simulink model "cuurent_controlled_circuit"  (R2022a)
settings: Solver=VariableStepAuto  StartTime=0.0  StopTime=25.0  RelTol=1e-3
undefined symbols (not defined in the file or in its folder): DiscIntNeverNeededParam
libraries: fl_lib x82, nesl_utility x65, eeRmsMeasurement x34, eePowerMeasurement x17, ee_lib x16
(part 1 of 3)
settings Model: Creator=qwxt1  LastModifiedBy=qwxt1

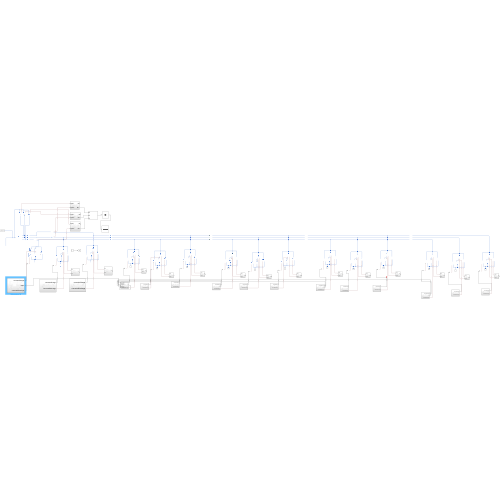
[thumbnail: Simulink's stored preview of the top-level diagram]
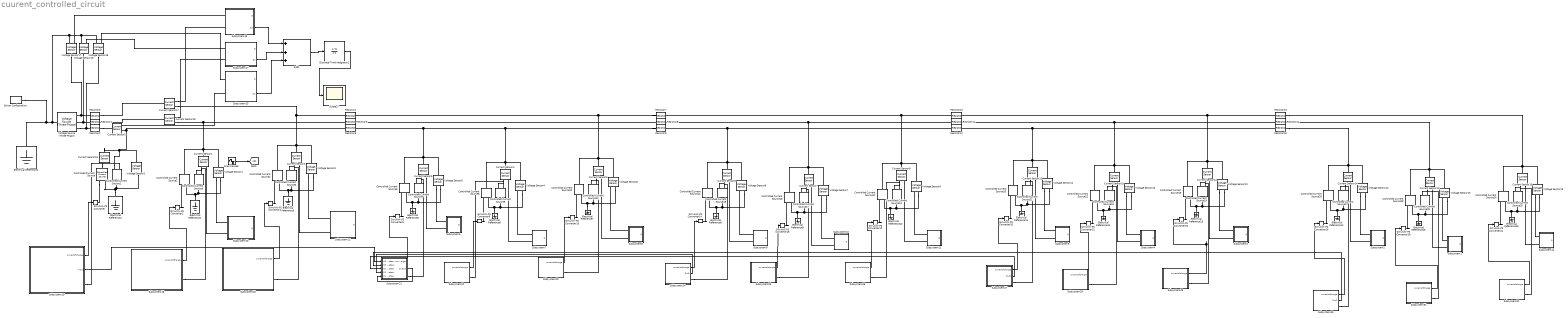
== system cuurent_controlled_circuit ==
  Add1 : Sum  Inputs=+++
  Controlled Current Source{,1..29} (30 alike) : fl_lib/Electrical/Electrical Sources/Controlled Current Source
      settings: SourceProductBaseCode=PW,SS,VE
  Current Sensor{1..17,19} (18 alike) : fl_lib/Electrical/Electrical Sensors/Current Sensor
      settings: SourceProductBaseCode=PW,SS,VE
  Discrete-Time Integrator2 : DiscreteIntegrator  InitialCondition=1500000  ICPrevOutput=DiscIntNeverNeededParam  ICPrevScaledInput=DiscIntNeverNeededParam
  Electrical Reference{1..16} (16 alike) : fl_lib/Electrical/Electrical Elements/Electrical Reference
      settings: SourceProductBaseCode=PW,SS,VE
  Goto : Goto
  Resistor1 : ee_lib/Passive/Resistor  R=0.01989 Ohm  enable_R_tol=0  R_tol=5  tol_distribution=1  nSigma=4  enable_operating_limits=0  operating_limit_action=2  max_working_voltage=100 V  power_rating=1 W  enable_faults=0  fault_action=1  R_faulted=inf Ohm  enable_temporal_fault=0  t_fault=1 s  enable_behavioral_fault=0  max_permissible_current=1 A  t_fail_on_current=1 s  noise_mode=0  sample_time=1e-3 s  repeatability=1  auto_seed=2915145293  user_seed=0  Tdevice=25 degC  power_derating_T1=70 degC  power_derating_T2=155 degC  operating_temperature_range_vec=[-50, 150] degC  alpha=3.93e-3 1/K  Tmeas=25 degC  thermal_mass=100 J/K  temperature_specify=off  temperature_priority=High  temperature=298.15 K  temperature_nominal_specify=off  temperature_nominal_unit=K  temperature_nominal_value=1
  Resistor10 : ee_lib/Passive/Resistor  R=0.040716 Ohm  enable_R_tol=0  R_tol=5  tol_distribution=1  nSigma=4  enable_operating_limits=0  operating_limit_action=2  max_working_voltage=100 V  power_rating=1 W  enable_faults=0  fault_action=1  R_faulted=inf Ohm  enable_temporal_fault=0  t_fault=1 s  enable_behavioral_fault=0  max_permissible_current=1 A  t_fail_on_current=1 s  noise_mode=0  sample_time=1e-3 s  repeatability=1  auto_seed=2513705850  user_seed=0  Tdevice=25 degC  power_derating_T1=70 degC  power_derating_T2=155 degC  operating_temperature_range_vec=[-50, 150] degC  alpha=3.93e-3 1/K  Tmeas=25 degC  thermal_mass=100 J/K  temperature_specify=off  temperature_priority=High  temperature=298.15 K  temperature_nominal_specify=off  temperature_nominal_unit=K  temperature_nominal_value=1
  Resistor11 : ee_lib/Passive/Resistor  R=0.040716 Ohm  enable_R_tol=0  R_tol=5  tol_distribution=1  nSigma=4  enable_operating_limits=0  operating_limit_action=2  max_working_voltage=100 V  power_rating=1 W  enable_faults=0  fault_action=1  R_faulted=inf Ohm  enable_temporal_fault=0  t_fault=1 s  enable_behavioral_fault=0  max_permissible_current=1 A  t_fail_on_current=1 s  noise_mode=0  sample_time=1e-3 s  repeatability=1  auto_seed=961264961  user_seed=0  Tdevice=25 degC  power_derating_T1=70 degC  power_derating_T2=155 degC  operating_temperature_range_vec=[-50, 150] degC  alpha=3.93e-3 1/K  Tmeas=25 degC  thermal_mass=100 J/K  temperature_specify=off  temperature_priority=High  temperature=298.15 K  temperature_nominal_specify=off  temperature_nominal_unit=K  temperature_nominal_value=1
  Resistor12 : ee_lib/Passive/Resistor  R=0.040716 Ohm  enable_R_tol=0  R_tol=5  tol_distribution=1  nSigma=4  enable_operating_limits=0  operating_limit_action=2  max_working_voltage=100 V  power_rating=1 W  enable_faults=0  fault_action=1  R_faulted=inf Ohm  enable_temporal_fault=0  t_fault=1 s  enable_behavioral_fault=0  max_permissible_current=1 A  t_fail_on_current=1 s  noise_mode=0  sample_time=1e-3 s  repeatability=1  auto_seed=3226667450  user_seed=0  Tdevice=25 degC  power_derating_T1=70 degC  power_derating_T2=155 degC  operating_temperature_range_vec=[-50, 150] degC  alpha=3.93e-3 1/K  Tmeas=25 degC  thermal_mass=100 J/K  temperature_specify=off  temperature_priority=High  temperature=298.15 K  temperature_nominal_specify=off  temperature_nominal_unit=K  temperature_nominal_value=1
  Resistor13 : ee_lib/Passive/Resistor  R=0.04524 Ohm  enable_R_tol=0  R_tol=5  tol_distribution=1  nSigma=4  enable_operating_limits=0  operating_limit_action=2  max_working_voltage=100 V  power_rating=1 W  enable_faults=0  fault_action=1  R_faulted=inf Ohm  enable_temporal_fault=0  t_fault=1 s  enable_behavioral_fault=0  max_permissible_current=1 A  t_fail_on_current=1 s  noise_mode=0  sample_time=1e-3 s  repeatability=1  auto_seed=1095625179  user_seed=0  Tdevice=25 degC  power_derating_T1=70 degC  power_derating_T2=155 degC  operating_temperature_range_vec=[-50, 150] degC  alpha=3.93e-3 1/K  Tmeas=25 degC  thermal_mass=100 J/K  temperature_specify=off  temperature_priority=High  temperature=298.15 K  temperature_nominal_specify=off  temperature_nominal_unit=K  temperature_nominal_value=1
  Resistor14 : ee_lib/Passive/Resistor  R=0.04524 Ohm  enable_R_tol=0  R_tol=5  tol_distribution=1  nSigma=4  enable_operating_limits=0  operating_limit_action=2  max_working_voltage=100 V  power_rating=1 W  enable_faults=0  fault_action=1  R_faulted=inf Ohm  enable_temporal_fault=0  t_fault=1 s  enable_behavioral_fault=0  max_permissible_current=1 A  t_fail_on_current=1 s  noise_mode=0  sample_time=1e-3 s  repeatability=1  auto_seed=2173068990  user_seed=0  Tdevice=25 degC  power_derating_T1=70 degC  power_derating_T2=155 degC  operating_temperature_range_vec=[-50, 150] degC  alpha=3.93e-3 1/K  Tmeas=25 degC  thermal_mass=100 J/K  temperature_specify=off  temperature_priority=High  temperature=298.15 K  temperature_nominal_specify=off  temperature_nominal_unit=K  temperature_nominal_value=1
  Resistor15 : ee_lib/Passive/Resistor  R=0.04524 Ohm  enable_R_tol=0  R_tol=5  tol_distribution=1  nSigma=4  enable_operating_limits=0  operating_limit_action=2  max_working_voltage=100 V  power_rating=1 W  enable_faults=0  fault_action=1  R_faulted=inf Ohm  enable_temporal_fault=0  t_fault=1 s  enable_behavioral_fault=0  max_permissible_current=1 A  t_fail_on_current=1 s  noise_mode=0  sample_time=1e-3 s  repeatability=1  auto_seed=3002511661  user_seed=0  Tdevice=25 degC  power_derating_T1=70 degC  power_derating_T2=155 degC  operating_temperature_range_vec=[-50, 150] degC  alpha=3.93e-3 1/K  Tmeas=25 degC  thermal_mass=100 J/K  temperature_specify=off  temperature_priority=High  temperature=298.15 K  temperature_nominal_specify=off  temperature_nominal_unit=K  temperature_nominal_value=1
  Resistor2 : ee_lib/Passive/Resistor  R=0.01989 Ohm  enable_R_tol=0  R_tol=5  tol_distribution=1  nSigma=4  enable_operating_limits=0  operating_limit_action=2  max_working_voltage=100 V  power_rating=1 W  enable_faults=0  fault_action=1  R_faulted=inf Ohm  enable_temporal_fault=0  t_fault=1 s  enable_behavioral_fault=0  max_permissible_current=1 A  t_fail_on_current=1 s  noise_mode=0  sample_time=1e-3 s  repeatability=1  auto_seed=3922919431  user_seed=0  Tdevice=25 degC  power_derating_T1=70 degC  power_derating_T2=155 degC  operating_temperature_range_vec=[-50, 150] degC  alpha=3.93e-3 1/K  Tmeas=25 degC  thermal_mass=100 J/K  temperature_specify=off  temperature_priority=High  temperature=298.15 K  temperature_nominal_specify=off  temperature_nominal_unit=K  temperature_nominal_value=1
  Resistor3 : ee_lib/Passive/Resistor  R=0.01989 Ohm  enable_R_tol=0  R_tol=5  tol_distribution=1  nSigma=4  enable_operating_limits=0  operating_limit_action=2  max_working_voltage=100 V  power_rating=1 W  enable_faults=0  fault_action=1  R_faulted=inf Ohm  enable_temporal_fault=0  t_fault=1 s  enable_behavioral_fault=0  max_permissible_current=1 A  t_fail_on_current=1 s  noise_mode=0  sample_time=1e-3 s  repeatability=1  auto_seed=198304613  user_seed=0  Tdevice=25 degC  power_derating_T1=70 degC  power_derating_T2=155 degC  operating_temperature_range_vec=[-50, 150] degC  alpha=3.93e-3 1/K  Tmeas=25 degC  thermal_mass=100 J/K  temperature_specify=off  temperature_priority=High  temperature=298.15 K  temperature_nominal_specify=off  temperature_nominal_unit=K  temperature_nominal_value=1
  Resistor4 : ee_lib/Passive/Resistor  R=0.0459 Ohm  enable_R_tol=0  R_tol=5  tol_distribution=1  nSigma=4  enable_operating_limits=0  operating_limit_action=2  max_working_voltage=100 V  power_rating=1 W  enable_faults=0  fault_action=1  R_faulted=inf Ohm  enable_temporal_fault=0  t_fault=1 s  enable_behavioral_fault=0  max_permissible_current=1 A  t_fail_on_current=1 s  noise_mode=0  sample_time=1e-3 s  repeatability=1  auto_seed=2813624503  user_seed=0  Tdevice=25 degC  power_derating_T1=70 degC  power_derating_T2=155 degC  operating_temperature_range_vec=[-50, 150] degC  alpha=3.93e-3 1/K  Tmeas=25 degC  thermal_mass=100 J/K  temperature_specify=off  temperature_priority=High  temperature=298.15 K  temperature_nominal_specify=off  temperature_nominal_unit=K  temperature_nominal_value=1
  Resistor5 : ee_lib/Passive/Resistor  R=0.0459 Ohm  enable_R_tol=0  R_tol=5  tol_distribution=1  nSigma=4  enable_operating_limits=0  operating_limit_action=2  max_working_voltage=100 V  power_rating=1 W  enable_faults=0  fault_action=1  R_faulted=inf Ohm  enable_temporal_fault=0  t_fault=1 s  enable_behavioral_fault=0  max_permissible_current=1 A  t_fail_on_current=1 s  noise_mode=0  sample_time=1e-3 s  repeatability=1  auto_seed=698412085  user_seed=0  Tdevice=25 degC  power_derating_T1=70 degC  power_derating_T2=155 degC  operating_temperature_range_vec=[-50, 150] degC  alpha=3.93e-3 1/K  Tmeas=25 degC  thermal_mass=100 J/K  temperature_specify=off  temperature_priority=High  temperature=298.15 K  temperature_nominal_specify=off  temperature_nominal_unit=K  temperature_nominal_value=1
  Resistor6 : ee_lib/Passive/Resistor  R=0.0459 Ohm  enable_R_tol=0  R_tol=5  tol_distribution=1  nSigma=4  enable_operating_limits=0  operating_limit_action=2  max_working_voltage=100 V  power_rating=1 W  enable_faults=0  fault_action=1  R_faulted=inf Ohm  enable_temporal_fault=0  t_fault=1 s  enable_behavioral_fault=0  max_permissible_current=1 A  t_fail_on_current=1 s  noise_mode=0  sample_time=1e-3 s  repeatability=1  auto_seed=511091151  user_seed=0  Tdevice=25 degC  power_derating_T1=70 degC  power_derating_T2=155 degC  operating_temperature_range_vec=[-50, 150] degC  alpha=3.93e-3 1/K  Tmeas=25 degC  thermal_mass=100 J/K  temperature_specify=off  temperature_priority=High  temperature=298.15 K  temperature_nominal_specify=off  temperature_nominal_unit=K  temperature_nominal_value=1
  Resistor7 : ee_lib/Passive/Resistor  R=0.039585 Ohm  enable_R_tol=0  R_tol=5  tol_distribution=1  nSigma=4  enable_operating_limits=0  operating_limit_action=2  max_working_voltage=100 V  power_rating=1 W  enable_faults=0  fault_action=1  R_faulted=inf Ohm  enable_temporal_fault=0  t_fault=1 s  enable_behavioral_fault=0  max_permissible_current=1 A  t_fail_on_current=1 s  noise_mode=0  sample_time=1e-3 s  repeatability=1  auto_seed=2140457305  user_seed=0  Tdevice=25 degC  power_derating_T1=70 degC  power_derating_T2=155 degC  operating_temperature_range_vec=[-50, 150] degC  alpha=3.93e-3 1/K  Tmeas=25 degC  thermal_mass=100 J/K  temperature_specify=off  temperature_priority=High  temperature=298.15 K  temperature_nominal_specify=off  temperature_nominal_unit=K  temperature_nominal_value=1
  Resistor8 : ee_lib/Passive/Resistor  R=0.039585 Ohm  enable_R_tol=0  R_tol=5  tol_distribution=1  nSigma=4  enable_operating_limits=0  operating_limit_action=2  max_working_voltage=100 V  power_rating=1 W  enable_faults=0  fault_action=1  R_faulted=inf Ohm  enable_temporal_fault=0  t_fault=1 s  enable_behavioral_fault=0  max_permissible_current=1 A  t_fail_on_current=1 s  noise_mode=0  sample_time=1e-3 s  repeatability=1  auto_seed=4122068914  user_seed=0  Tdevice=25 degC  power_derating_T1=70 degC  power_derating_T2=155 degC  operating_temperature_range_vec=[-50, 150] degC  alpha=3.93e-3 1/K  Tmeas=25 degC  thermal_mass=100 J/K  temperature_specify=off  temperature_priority=High  temperature=298.15 K  temperature_nominal_specify=off  temperature_nominal_unit=K  temperature_nominal_value=1
  Resistor9 : ee_lib/Passive/Resistor  R=0.039585 Ohm  enable_R_tol=0  R_tol=5  tol_distribution=1  nSigma=4  enable_operating_limits=0  operating_limit_action=2  max_working_voltage=100 V  power_rating=1 W  enable_faults=0  fault_action=1  R_faulted=inf Ohm  enable_temporal_fault=0  t_fault=1 s  enable_behavioral_fault=0  max_permissible_current=1 A  t_fail_on_current=1 s  noise_mode=0  sample_time=1e-3 s  repeatability=1  auto_seed=1461945564  user_seed=0  Tdevice=25 degC  power_derating_T1=70 degC  power_derating_T2=155 degC  operating_temperature_range_vec=[-50, 150] degC  alpha=3.93e-3 1/K  Tmeas=25 degC  thermal_mass=100 J/K  temperature_specify=off  temperature_priority=High  temperature=298.15 K  temperature_nominal_specify=off  temperature_nominal_unit=K  temperature_nominal_value=1
  Scope27 : Scope
  Simulink-PS Converter{,2,4,6,8,10,12,14,16,18,20,22,24,26,28} (15 alike) : nesl_utility/Simulink-PS Converter  PhysicalDomain=network_engine_domain  SubClassName=ps_input  LeftPortType=input  RightPortType=output  PseudoPeriodic=off  Frequencies=[]  NoiseDistribution=none  NoiseParameters=[]  Unit=1  AffineConversion=off  FilteringAndDerivatives=provide  SimscapeFilterOrder=1  InputFilterTimeConstant=0.001  UdotUserProvided=0
      settings: SourceProductBaseCode=SS,PW,VE
  Sine Wave16 : Sin  Frequency=314.6  SampleTime=0
  Solver Configuration : nesl_utility/Solver Configuration  PhysicalDomain=network_engine_domain  SubClassName=solver  LeftPortType=input  RightPortType=generic  Tones=[]  Harmonics=[]  SimulateNoise=off  Profile=off  UseLocalSampling=off  EnableSwitchedLinearOptims=on  FrequencyDomain=off  UseCCode=off  RelTol=0.001  AbsTol=0.001  MinStep=1e-09  ToWorkspace=off  RevertToSquareIcSolve=off  NumHomotopyIterations=100  PhasorMode=off  PhasorModeNumHarmonics=1  IndexReductionMethod=DerivativeReplacement  DoDC=off  ResidualTolerance=1e-09  UseLocalSolver=off  LocalSolverChoice=NE_BACKWARD_EULER_ADVANCER  LocalSolverSampleTime=0.001  DoFixedCost=off  MaxNonlinIter=3  MaxModeIter=2  ComputeImpulses=off  ImpulseIterations=2  LinearAlgebra=auto  LinearAlgebraNumThread=0  EquationFormulation=NE_TIME_EF  DelaysMemoryBudget=1024  AutomaticFiltering=on  FilteringTimeConstant=0.001  PartitionStorageMethod=AS_NEEDED  PartitionMemoryBudget=1024  PartitionMethod=ROBUST
      settings: SourceProductBaseCode=SS,PW,VE
  Subsystem1 : Subsystem
  Subsystem10 : Subsystem
  Subsystem11 : Subsystem
  Subsystem12 : Subsystem
  Subsystem13 : Subsystem
  Subsystem14 : Subsystem
  Subsystem15 : Subsystem
  Subsystem16 : Subsystem
  Subsystem17 : Subsystem
  Subsystem18 : Subsystem
  Subsystem19 : Subsystem
  Subsystem2 : Subsystem
  Subsystem20 : Subsystem
  Subsystem21 : Subsystem
  Subsystem22 : Subsystem
  Subsystem23 : Subsystem
  Subsystem24 : Subsystem
  Subsystem25 : Subsystem
  Subsystem26 : Subsystem
  Subsystem27 : Subsystem
  Subsystem28 : Subsystem
  Subsystem29 : Subsystem
  Subsystem3 : Subsystem
  Subsystem30 : Subsystem
  Subsystem31 : Subsystem
  Subsystem32 : Subsystem
  Subsystem4 : Subsystem
  Subsystem5 : Subsystem
  Subsystem6 : Subsystem
  Subsystem7 : Subsystem
  Subsystem8 : Subsystem
  Subsystem9 : Subsystem
  Voltage Source (Three-Phase) : ee_lib/Sources/Voltage Source (Three-Phase)  vline_rms=400 V  shift=0 deg  freq=50 Hz  impedance_option=0  SShortCircuit=1e6 A*V  XR=15  R=0.01 Ohm  L=3.97e-4 H  harmonic_option=0  harmonic_orders=[5, 7, 11, 13]  harmonic_ratios=[.1, .1, .1, .1]  G_parasitic=0 1/Ohm  I_specify=off  I_priority=None  I=[0, 0, 0] A  I_nominal_specify=off  I_nominal_unit=A  I_nominal_value=1
      settings: SourceProductBaseCode=PS  InternalSimscapePortConfiguration="{\"Bottom\":[],\"Left\":[{\"id\":\"n\",\"label\":\"n\",\"type\":\"foundation.electrical.electrical\"}],\"Right\":[{\"id\":\"a\",\"label\":\"a\",\"type\":\"foundation.electrical.electrical\"},{\"id\":\"b\",\"label\":\"b\",\"type\":\"foundation.electrical.electrical\"},{\"id\":\"c\",\"label\":\"c\",\"type\":\"foundation.electrical.electrical\"}],\"Top\":[]}"
  Voltage Sensor{1..18} (18 alike) : fl_lib/Electrical/Electrical Sensors/Voltage Sensor
      settings: SourceProductBaseCode=PW,SS,VE
  wires:
  Subsystem28/1(currentofcharge) -> Simulink-PS Converter22/1
  Subsystem26/1(currentofcharge) -> Simulink-PS Converter12/1
  Subsystem24/1(currentofcharge) -> Simulink-PS Converter14/1
  Sine Wave16/1 -> Goto/1
  Add1/1 -> Discrete-Time Integrator2/1
  Discrete-Time Integrator2/1 -> Scope27/1
  Subsystem18/2(Q1) -> Add1/1
  Subsystem17/2(Q1) -> Add1/2
  Subsystem15/2(Q1) -> Add1/3
  Subsystem19/1(currentofcharge) -> Simulink-PS Converter/1
  Subsystem20/1(currentofcharge) -> Simulink-PS Converter4/1
  Subsystem30/1(currentofcharge) -> Simulink-PS Converter26/1
  Subsystem21/1(currentofcharge) -> Simulink-PS Converter6/1
  Subsystem22/1(currentofcharge) -> Simulink-PS Converter8/1
  Subsystem23/1(currentofcharge) -> Simulink-PS Converter10/1
  Subsystem25/1(currentofcharge) -> Simulink-PS Converter16/1
  Subsystem27/1(currentofcharge) -> Simulink-PS Converter20/1
  Subsystem29/1(currentofcharge) -> Simulink-PS Converter18/1
  Subsystem31/1(currentofcharge) -> Simulink-PS Converter28/1
  Subsystem32/1(currentofcharge) -> Simulink-PS Converter24/1
  Subsystem16/1(currentofcharge) -> Simulink-PS Converter2/1
  Subsystem19/2(Input) -> Subsystem21/1(M5 Battery)
  Subsystem24/2(Out2) -> Subsystem21/4(M2 Battery)
  Subsystem27/2(Out2) -> Subsystem21/3(M1 Battery)
  Subsystem30/2(Out2) -> Subsystem21/2(M3 Battery)
  Subsystem21/2(Output) -> Subsystem21/5(M4 Battery)
  connections:
  Resistor3/LConn1 -- Voltage Sensor17/LConn1 -- Voltage Source (Three-Phase)/RConn1
  Resistor1/LConn1 -- Voltage Sensor16/LConn1 -- Voltage Source (Three-Phase)/RConn2
  Voltage Source (Three-Phase)/RConn3 -- Voltage Sensor18/LConn1 -- Resistor2/LConn1
  Voltage Sensor3/LConn1 -- Current Sensor17/RConn2 -- Resistor4/LConn1 -- Current Sensor3/LConn1 -- Controlled Current Source4/LConn1
  Resistor6/LConn1 -- Controlled Current Source1/RConn2 -- Current Sensor16/LConn1 -- Voltage Sensor2/LConn1 -- Current Sensor2/RConn2
  Subsystem15/LConn2 -- Current Sensor2/RConn1
  Voltage Sensor1/LConn1 -- Resistor5/LConn1 -- Current Sensor19/RConn2 -- Current Sensor1/LConn1 -- Controlled Current Source2/LConn1
  Electrical Reference4/LConn1 -- Voltage Sensor18/RConn2 -- Voltage Sensor16/RConn2 -- Voltage Sensor17/RConn2 -- Voltage Source (Three-Phase)/LConn1 -- Solver Configuration/RConn1
  Voltage Sensor9/LConn1 -- Resistor10/LConn1 -- Resistor7/RConn1 -- Current Sensor9/LConn1 -- Controlled Current Source12/LConn1
  Resistor8/LConn1 -- Resistor5/RConn1
  Voltage Sensor8/LConn1 -- Resistor12/LConn1 -- Resistor9/RConn1 -- Current Sensor8/LConn1 -- Controlled Current Source14/LConn1
  Voltage Sensor6/LConn1 -- Resistor7/LConn1 -- Resistor4/RConn1 -- Current Sensor6/LConn1 -- Controlled Current Source10/LConn1
  Voltage Sensor7/LConn1 -- Resistor11/LConn1 -- Resistor8/RConn1 -- Current Sensor7/LConn1 -- Controlled Current Source16/LConn1
  Voltage Sensor4/LConn1 -- Resistor9/LConn1 -- Voltage Sensor5/LConn1 -- Current Sensor5/LConn1 -- Controlled Current Source6/LConn1 -- Resistor6/RConn1 -- Current Sensor4/LConn1 -- Controlled Current Source8/LConn1
  Voltage Sensor12/LConn1 -- Resistor13/LConn1 -- Resistor10/RConn1 -- Current Sensor12/LConn1 -- Controlled Current Source18/LConn1
  Voltage Sensor10/LConn1 -- Resistor14/LConn1 -- Resistor11/RConn1 -- Current Sensor10/LConn1 -- Controlled Current Source22/LConn1
  Voltage Sensor11/LConn1 -- Resistor15/LConn1 -- Resistor12/RConn1 -- Current Sensor11/LConn1 -- Controlled Current Source20/LConn1
  Electrical Reference2/LConn1 -- Controlled Current Source2/RConn2 -- Voltage Sensor1/RConn2 -- Controlled Current Source3/LConn1
  Voltage Sensor1/RConn1 -- Subsystem13/LConn1
  Simulink-PS Converter2/RConn1 -- Controlled Current Source2/RConn1
  Current Sensor1/RConn1 -- Subsystem13/LConn2
  Current Sensor1/RConn2 -- Controlled Current Source3/RConn2
  Electrical Reference3/LConn1 -- Controlled Current Source4/RConn2 -- Voltage Sensor3/RConn2 -- Controlled Current Source5/LConn1
  Voltage Sensor3/RConn1 -- Subsystem12/LConn1
  Simulink-PS Converter4/RConn1 -- Controlled Current Source4/RConn1
  Current Sensor3/RConn1 -- Subsystem12/LConn2
  Current Sensor3/RConn2 -- Controlled Current Source5/RConn2
  Electrical Reference6/LConn1 -- Voltage Sensor4/RConn2 -- Controlled Current Source9/LConn1 -- Controlled Current Source8/RConn2
  Electrical Reference7/LConn1 -- Voltage Sensor6/RConn2 -- Controlled Current Source11/LConn1 -- Controlled Current Source10/RConn2
  Electrical Reference5/LConn1 -- Voltage Sensor5/RConn2 -- Controlled Current Source7/LConn1 -- Controlled Current Source6/RConn2
  Simulink-PS Converter6/RConn1 -- Controlled Current Source6/RConn1
  Simulink-PS Converter8/RConn1 -- Controlled Current Source8/RConn1
  Subsystem8/LConn2 -- Current Sensor6/RConn1
  Current Sensor4/RConn2 -- Controlled Current Source9/RConn2
  Subsystem7/LConn1 -- Voltage Sensor4/RConn1
  Current Sensor6/RConn2 -- Controlled Current Source11/RConn2
  Subsystem8/LConn1 -- Voltage Sensor6/RConn1
  Simulink-PS Converter10/RConn1 -- Controlled Current Source10/RConn1
  Current Sensor5/RConn1 -- Subsystem6/LConn2
  Subsystem7/LConn2 -- Current Sensor4/RConn1
  Current Sensor5/RConn2 -- Controlled Current Source7/RConn2
  Controlled Current Source15/LConn1 -- Voltage Sensor8/RConn2 -- Controlled Current Source14/RConn2 -- Electrical Reference8/LConn1
  Controlled Current Source13/LConn1 -- Voltage Sensor9/RConn2 -- Controlled Current Source12/RConn2 -- Electrical Reference10/LConn1
  Controlled Current Source17/LConn1 -- Voltage Sensor7/RConn2 -- Controlled Current Source16/RConn2 -- Electrical Reference9/LConn1
  Simulink-PS Converter12/RConn1 -- Controlled Current Source12/RConn1
  Current Sensor9/RConn2 -- Controlled Current Source13/RConn2
  Simulink-PS Converter16/RConn1 -- Controlled Current Source16/RConn1
  Subsystem9/LConn1 -- Voltage Sensor8/RConn1
  Subsystem11/LConn2 -- Current Sensor9/RConn1
  Current Sensor7/RConn2 -- Controlled Current Source17/RConn2
  Subsystem10/LConn1 -- Voltage Sensor7/RConn1
  Subsystem10/LConn2 -- Current Sensor7/RConn1
  Subsystem9/LConn2 -- Current Sensor8/RConn1
  Current Sensor8/RConn2 -- Controlled Current Source15/RConn2
  Simulink-PS Converter14/RConn1 -- Controlled Current Source14/RConn1
  Subsystem11/LConn1 -- Voltage Sensor9/RConn1
  Controlled Current Source21/LConn1 -- Voltage Sensor11/RConn2 -- Controlled Current Source20/RConn2 -- Electrical Reference11/LConn1
  Controlled Current Source19/LConn1 -- Voltage Sensor12/RConn2 -- Controlled Current Source18/RConn2 -- Electrical Reference13/LConn1
  Controlled Current Source23/LConn1 -- Voltage Sensor10/RConn2 -- Controlled Current Source22/RConn2 -- Electrical Reference12/LConn1
  Simulink-PS Converter18/RConn1 -- Controlled Current Source18/RConn1
  Current Sensor12/RConn2 -- Controlled Current Source19/RConn2
  Simulink-PS Converter22/RConn1 -- Controlled Current Source22/RConn1
  Voltage Sensor11/RConn1 -- Subsystem5/LConn1
  Current Sensor12/RConn1 -- Subsystem3/LConn2
  Current Sensor10/RConn2 -- Controlled Current Source23/RConn2
  Voltage Sensor10/RConn1 -- Subsystem4/LConn1
  Current Sensor10/RConn1 -- Subsystem4/LConn2
  Current Sensor11/RConn1 -- Subsystem5/LConn2
  Current Sensor11/RConn2 -- Controlled Current Source21/RConn2
  Simulink-PS Converter20/RConn1 -- Controlled Current Source20/RConn1
  Voltage Sensor12/RConn1 -- Subsystem3/LConn1
  Voltage Sensor13/LConn1 -- Resistor14/RConn1 -- Current Sensor13/LConn1 -- Controlled Current Source28/LConn1
  Controlled Current Source27/LConn1 -- Voltage Sensor14/RConn2 -- Controlled Current Source26/RConn2 -- Electrical Reference14/LConn1
  Controlled Current Source25/LConn1 -- Voltage Sensor15/RConn2 -- Controlled Current Source24/RConn2 -- Electrical Reference16/LConn1
  Controlled Current Source29/LConn1 -- Voltage Sensor13/RConn2 -- Controlled Current Source28/RConn2 -- Electrical Reference15/LConn1
  Voltage Sensor15/LConn1 -- Resistor13/RConn1 -- Current Sensor15/LConn1 -- Controlled Current Source24/LConn1
  Voltage Sensor14/LConn1 -- Resistor15/RConn1 -- Current Sensor14/LConn1 -- Controlled Current Source26/LConn1
  Simulink-PS Converter24/RConn1 -- Controlled Current Source24/RConn1
  Current Sensor15/RConn2 -- Controlled Current Source25/RConn2
  Simulink-PS Converter28/RConn1 -- Controlled Current Source28/RConn1
  Voltage Sensor14/RConn1 -- Subsystem2/LConn1
  Current Sensor15/RConn1 -- Subsystem14/LConn2
  Current Sensor13/RConn2 -- Controlled Current Source29/RConn2
  Subsystem1/LConn1 -- Voltage Sensor13/RConn1
  Subsystem1/LConn2 -- Current Sensor13/RConn1
  Current Sensor14/RConn1 -- Subsystem2/LConn2
  Current Sensor14/RConn2 -- Controlled Current Source27/RConn2
  Simulink-PS Converter26/RConn1 -- Controlled Current Source26/RConn1
  Voltage Sensor15/RConn1 -- Subsystem14/LConn1
  Current Sensor16/RConn2 -- Controlled Current Source/LConn1
  Controlled Current Source/RConn1 -- Simulink-PS Converter/RConn1
  Resistor2/RConn1 -- Current Sensor2/LConn1
  Voltage Sensor5/RConn1 -- Subsystem6/LConn1
  Electrical Reference1/LConn1 -- Controlled Current Source/RConn2 -- Voltage Sensor2/RConn2 -- Controlled Current Source1/LConn1
  Resistor1/RConn1 -- Current Sensor19/LConn1
  Resistor3/RConn1 -- Current Sensor17/LConn1
  Current Sensor19/RConn1 -- Subsystem17/LConn2
  Current Sensor17/RConn1 -- Subsystem18/LConn2
  Voltage Sensor17/RConn1 -- Subsystem18/LConn1
  Voltage Sensor18/RConn1 -- Subsystem15/LConn1
  Voltage Sensor16/RConn1 -- Subsystem17/LConn1
  Subsystem19/RConn1 -- Controlled Current Source1/RConn1
  Subsystem20/RConn1 -- Controlled Current Source5/RConn1
  Subsystem30/RConn1 -- Controlled Current Source27/RConn1
  Subsystem21/RConn1 -- Controlled Current Source7/RConn1
  Subsystem23/RConn1 -- Controlled Current Source11/RConn1
  Subsystem24/RConn1 -- Controlled Current Source15/RConn1
  Subsystem25/RConn1 -- Controlled Current Source17/RConn1
  Subsystem26/RConn1 -- Controlled Current Source13/RConn1
  Subsystem27/RConn1 -- Controlled Current Source21/RConn1
  Subsystem28/RConn1 -- Controlled Current Source23/RConn1
  Subsystem29/RConn1 -- Controlled Current Source19/RConn1
  Subsystem31/RConn1 -- Controlled Current Source29/RConn1
  Subsystem32/RConn1 -- Controlled Current Source25/RConn1
  Subsystem16/RConn1 -- Controlled Current Source3/RConn1
  Subsystem22/RConn1 -- Controlled Current Source9/RConn1

== system cuurent_controlled_circuit/Subsystem1 ==
  Display3 : Display
  Display4 : Display
  Display5 : Display
  PS-Simulink Converter2 : nesl_utility/PS-Simulink Converter  PhysicalDomain=network_engine_domain  SubClassName=ps_output  LeftPortType=input  RightPortType=output  PseudoPeriodic=off  Frequencies=[]  VectorFormat=inherit  Unit=inherit  AffineConversion=off
      settings: SourceProductBaseCode=SS,PW,VE
  PS-Simulink Converter3 : nesl_utility/PS-Simulink Converter  PhysicalDomain=network_engine_domain  SubClassName=ps_output  LeftPortType=input  RightPortType=output  PseudoPeriodic=off  Frequencies=[]  VectorFormat=inherit  Unit=inherit  AffineConversion=off
      settings: SourceProductBaseCode=SS,PW,VE
  Power Measurement2 : eePowerMeasurement/Power Measurement  LabelModeActiveChoice=Continuous  F=50  K=[0 1 2 3]  Ts=0
      settings: SourceProductBaseCode=PS
  RMS Measurement2 : eeRmsMeasurement/RMS Measurement  LabelModeActiveChoice=Total  F=50  SpecifyHarmonics=off  K=[0 1 2]  Ts=0
      settings: SourceProductBaseCode=PS
  RMS Measurement3 : eeRmsMeasurement/RMS Measurement  LabelModeActiveChoice=Total  F=50  SpecifyHarmonics=off  K=[0 1 2]  Ts=0
      settings: SourceProductBaseCode=PS
  Scope{6..10} (5 alike) : Scope
  input : PMIOPort  Side=Left
  input1 : PMIOPort  Port=2  Side=Left
  Q : Outport
  wires:
  Power Measurement2/2 -> Q/1
  PS-Simulink Converter3/1 -> RMS Measurement3/1, Scope8/1
  Power Measurement2/1 -> Display5/1, Scope10/1
  RMS Measurement2/1 -> Scope7/1, Display3/1, Power Measurement2/1
  PS-Simulink Converter2/1 -> RMS Measurement2/1, Scope6/1
  RMS Measurement3/1 -> Power Measurement2/2, Scope9/1, Display4/1
  connections:
  PS-Simulink Converter3/LConn1 -- input1/RConn1
  PS-Simulink Converter2/LConn1 -- input/RConn1

== system cuurent_controlled_circuit/Subsystem10 ==
  Display3 : Display
  Display4 : Display
  Display5 : Display
  PS-Simulink Converter2 : nesl_utility/PS-Simulink Converter  PhysicalDomain=network_engine_domain  SubClassName=ps_output  LeftPortType=input  RightPortType=output  PseudoPeriodic=off  Frequencies=[]  VectorFormat=inherit  Unit=inherit  AffineConversion=off
      settings: SourceProductBaseCode=SS,PW,VE
  PS-Simulink Converter3 : nesl_utility/PS-Simulink Converter  PhysicalDomain=network_engine_domain  SubClassName=ps_output  LeftPortType=input  RightPortType=output  PseudoPeriodic=off  Frequencies=[]  VectorFormat=inherit  Unit=inherit  AffineConversion=off
      settings: SourceProductBaseCode=SS,PW,VE
  Power Measurement2 : eePowerMeasurement/Power Measurement  LabelModeActiveChoice=Continuous  F=50  K=[0 1 2 3]  Ts=0
      settings: SourceProductBaseCode=PS
  RMS Measurement2 : eeRmsMeasurement/RMS Measurement  LabelModeActiveChoice=Total  F=50  SpecifyHarmonics=off  K=[0 1 2]  Ts=0
      settings: SourceProductBaseCode=PS
  RMS Measurement3 : eeRmsMeasurement/RMS Measurement  LabelModeActiveChoice=Total  F=50  SpecifyHarmonics=off  K=[0 1 2]  Ts=0
      settings: SourceProductBaseCode=PS
  Scope{6..10} (5 alike) : Scope
  input : PMIOPort  Side=Left
  input1 : PMIOPort  Port=2  Side=Left
  Q : Outport
  wires:
  Power Measurement2/2 -> Q/1
  PS-Simulink Converter3/1 -> RMS Measurement3/1, Scope8/1
  Power Measurement2/1 -> Display5/1, Scope10/1
  RMS Measurement2/1 -> Scope7/1, Display3/1, Power Measurement2/1
  PS-Simulink Converter2/1 -> RMS Measurement2/1, Scope6/1
  RMS Measurement3/1 -> Power Measurement2/2, Scope9/1, Display4/1
  connections:
  PS-Simulink Converter3/LConn1 -- input1/RConn1
  PS-Simulink Converter2/LConn1 -- input/RConn1

== system cuurent_controlled_circuit/Subsystem11 ==
  Display3 : Display
  Display4 : Display
  Display5 : Display
  PS-Simulink Converter2 : nesl_utility/PS-Simulink Converter  PhysicalDomain=network_engine_domain  SubClassName=ps_output  LeftPortType=input  RightPortType=output  PseudoPeriodic=off  Frequencies=[]  VectorFormat=inherit  Unit=inherit  AffineConversion=off
      settings: SourceProductBaseCode=SS,PW,VE
  PS-Simulink Converter3 : nesl_utility/PS-Simulink Converter  PhysicalDomain=network_engine_domain  SubClassName=ps_output  LeftPortType=input  RightPortType=output  PseudoPeriodic=off  Frequencies=[]  VectorFormat=inherit  Unit=inherit  AffineConversion=off
      settings: SourceProductBaseCode=SS,PW,VE
  Power Measurement2 : eePowerMeasurement/Power Measurement  LabelModeActiveChoice=Continuous  F=50  K=[0 1 2 3]  Ts=0
      settings: SourceProductBaseCode=PS
  RMS Measurement2 : eeRmsMeasurement/RMS Measurement  LabelModeActiveChoice=Total  F=50  SpecifyHarmonics=off  K=[0 1 2]  Ts=0
      settings: SourceProductBaseCode=PS
  RMS Measurement3 : eeRmsMeasurement/RMS Measurement  LabelModeActiveChoice=Total  F=50  SpecifyHarmonics=off  K=[0 1 2]  Ts=0
      settings: SourceProductBaseCode=PS
  Scope{6..10} (5 alike) : Scope
  input : PMIOPort  Side=Left
  input1 : PMIOPort  Port=2  Side=Left
  Q : Outport
  wires:
  Power Measurement2/2 -> Q/1
  PS-Simulink Converter3/1 -> RMS Measurement3/1, Scope8/1
  Power Measurement2/1 -> Display5/1, Scope10/1
  RMS Measurement2/1 -> Scope7/1, Display3/1, Power Measurement2/1
  PS-Simulink Converter2/1 -> RMS Measurement2/1, Scope6/1
  RMS Measurement3/1 -> Power Measurement2/2, Scope9/1, Display4/1
  connections:
  PS-Simulink Converter3/LConn1 -- input1/RConn1
  PS-Simulink Converter2/LConn1 -- input/RConn1

== system cuurent_controlled_circuit/Subsystem12 ==
  Display3 : Display
  Display4 : Display
  Display5 : Display
  PS-Simulink Converter2 : nesl_utility/PS-Simulink Converter  PhysicalDomain=network_engine_domain  SubClassName=ps_output  LeftPortType=input  RightPortType=output  PseudoPeriodic=off  Frequencies=[]  VectorFormat=inherit  Unit=inherit  AffineConversion=off
      settings: SourceProductBaseCode=SS,PW,VE
  PS-Simulink Converter3 : nesl_utility/PS-Simulink Converter  PhysicalDomain=network_engine_domain  SubClassName=ps_output  LeftPortType=input  RightPortType=output  PseudoPeriodic=off  Frequencies=[]  VectorFormat=inherit  Unit=inherit  AffineConversion=off
      settings: SourceProductBaseCode=SS,PW,VE
  Power Measurement2 : eePowerMeasurement/Power Measurement  LabelModeActiveChoice=Continuous  F=50  K=[0 1 2 3]  Ts=0
      settings: SourceProductBaseCode=PS
  RMS Measurement2 : eeRmsMeasurement/RMS Measurement  LabelModeActiveChoice=Total  F=50  SpecifyHarmonics=off  K=[0 1 2]  Ts=0
      settings: SourceProductBaseCode=PS
  RMS Measurement3 : eeRmsMeasurement/RMS Measurement  LabelModeActiveChoice=Total  F=50  SpecifyHarmonics=off  K=[0 1 2]  Ts=0
      settings: SourceProductBaseCode=PS
  Scope{6..10} (5 alike) : Scope
  input : PMIOPort  Side=Left
  input1 : PMIOPort  Port=2  Side=Left
  Q : Outport
  wires:
  Power Measurement2/2 -> Q/1
  PS-Simulink Converter3/1 -> RMS Measurement3/1, Scope8/1
  Power Measurement2/1 -> Display5/1, Scope10/1
  RMS Measurement2/1 -> Scope7/1, Display3/1, Power Measurement2/1
  PS-Simulink Converter2/1 -> RMS Measurement2/1, Scope6/1
  RMS Measurement3/1 -> Power Measurement2/2, Scope9/1, Display4/1
  connections:
  PS-Simulink Converter3/LConn1 -- input1/RConn1
  PS-Simulink Converter2/LConn1 -- input/RConn1

== system cuurent_controlled_circuit/Subsystem13 ==
  Display3 : Display
  Display4 : Display
  Display5 : Display
  PS-Simulink Converter2 : nesl_utility/PS-Simulink Converter  PhysicalDomain=network_engine_domain  SubClassName=ps_output  LeftPortType=input  RightPortType=output  PseudoPeriodic=off  Frequencies=[]  VectorFormat=inherit  Unit=inherit  AffineConversion=off
      settings: SourceProductBaseCode=SS,PW,VE
  PS-Simulink Converter3 : nesl_utility/PS-Simulink Converter  PhysicalDomain=network_engine_domain  SubClassName=ps_output  LeftPortType=input  RightPortType=output  PseudoPeriodic=off  Frequencies=[]  VectorFormat=inherit  Unit=inherit  AffineConversion=off
      settings: SourceProductBaseCode=SS,PW,VE
  Power Measurement2 : eePowerMeasurement/Power Measurement  LabelModeActiveChoice=Continuous  F=50  K=[0 1 2 3]  Ts=0
      settings: SourceProductBaseCode=PS
  RMS Measurement2 : eeRmsMeasurement/RMS Measurement  LabelModeActiveChoice=Total  F=50  SpecifyHarmonics=off  K=[0 1 2]  Ts=0
      settings: SourceProductBaseCode=PS
  RMS Measurement3 : eeRmsMeasurement/RMS Measurement  LabelModeActiveChoice=Total  F=50  SpecifyHarmonics=off  K=[0 1 2]  Ts=0
      settings: SourceProductBaseCode=PS
  Scope{6..10} (5 alike) : Scope
  input : PMIOPort  Side=Left
  input1 : PMIOPort  Port=2  Side=Left
  Q : Outport
  wires:
  Power Measurement2/2 -> Q/1
  PS-Simulink Converter3/1 -> RMS Measurement3/1, Scope8/1
  Power Measurement2/1 -> Display5/1, Scope10/1
  RMS Measurement2/1 -> Scope7/1, Display3/1, Power Measurement2/1
  PS-Simulink Converter2/1 -> RMS Measurement2/1, Scope6/1
  RMS Measurement3/1 -> Power Measurement2/2, Scope9/1, Display4/1
  connections:
  PS-Simulink Converter3/LConn1 -- input1/RConn1
  PS-Simulink Converter2/LConn1 -- input/RConn1

== system cuurent_controlled_circuit/Subsystem14 ==
  Display3 : Display
  Display4 : Display
  Display5 : Display
  PS-Simulink Converter2 : nesl_utility/PS-Simulink Converter  PhysicalDomain=network_engine_domain  SubClassName=ps_output  LeftPortType=input  RightPortType=output  PseudoPeriodic=off  Frequencies=[]  VectorFormat=inherit  Unit=inherit  AffineConversion=off
      settings: SourceProductBaseCode=SS,PW,VE
  PS-Simulink Converter3 : nesl_utility/PS-Simulink Converter  PhysicalDomain=network_engine_domain  SubClassName=ps_output  LeftPortType=input  RightPortType=output  PseudoPeriodic=off  Frequencies=[]  VectorFormat=inherit  Unit=inherit  AffineConversion=off
      settings: SourceProductBaseCode=SS,PW,VE
  Power Measurement2 : eePowerMeasurement/Power Measurement  LabelModeActiveChoice=Continuous  F=50  K=[0 1 2 3]  Ts=0
      settings: SourceProductBaseCode=PS
  RMS Measurement2 : eeRmsMeasurement/RMS Measurement  LabelModeActiveChoice=Total  F=50  SpecifyHarmonics=off  K=[0 1 2]  Ts=0
      settings: SourceProductBaseCode=PS
  RMS Measurement3 : eeRmsMeasurement/RMS Measurement  LabelModeActiveChoice=Total  F=50  SpecifyHarmonics=off  K=[0 1 2]  Ts=0
      settings: SourceProductBaseCode=PS
  Scope{6..10} (5 alike) : Scope
  input : PMIOPort  Side=Left
  input1 : PMIOPort  Port=2  Side=Left
  Q : Outport
  wires:
  Power Measurement2/2 -> Q/1
  PS-Simulink Converter3/1 -> RMS Measurement3/1, Scope8/1
  Power Measurement2/1 -> Display5/1, Scope10/1
  RMS Measurement2/1 -> Scope7/1, Display3/1, Power Measurement2/1
  PS-Simulink Converter2/1 -> RMS Measurement2/1, Scope6/1
  RMS Measurement3/1 -> Power Measurement2/2, Scope9/1, Display4/1
  connections:
  PS-Simulink Converter3/LConn1 -- input1/RConn1
  PS-Simulink Converter2/LConn1 -- input/RConn1

== system cuurent_controlled_circuit/Subsystem15 ==
  Display3 : Display
  Display4 : Display
  Display5 : Display
  PS-Simulink Converter2 : nesl_utility/PS-Simulink Converter  PhysicalDomain=network_engine_domain  SubClassName=ps_output  LeftPortType=input  RightPortType=output  PseudoPeriodic=off  Frequencies=[]  VectorFormat=inherit  Unit=inherit  AffineConversion=off
      settings: SourceProductBaseCode=SS,PW,VE
  PS-Simulink Converter3 : nesl_utility/PS-Simulink Converter  PhysicalDomain=network_engine_domain  SubClassName=ps_output  LeftPortType=input  RightPortType=output  PseudoPeriodic=off  Frequencies=[]  VectorFormat=inherit  Unit=inherit  AffineConversion=off
      settings: SourceProductBaseCode=SS,PW,VE
  Power Measurement2 : eePowerMeasurement/Power Measurement  LabelModeActiveChoice=Continuous  F=50  K=[0 1 2 3]  Ts=0
      settings: SourceProductBaseCode=PS
  RMS Measurement2 : eeRmsMeasurement/RMS Measurement  LabelModeActiveChoice=Total  F=50  SpecifyHarmonics=off  K=[0 1 2]  Ts=0
      settings: SourceProductBaseCode=PS
  RMS Measurement3 : eeRmsMeasurement/RMS Measurement  LabelModeActiveChoice=Total  F=50  SpecifyHarmonics=off  K=[0 1 2]  Ts=0
      settings: SourceProductBaseCode=PS
  Scope{6..10} (5 alike) : Scope
  input : PMIOPort  Side=Left
  input1 : PMIOPort  Port=2  Side=Left
  Q : Outport
  Q1 : Outport  Port=2
  wires:
  Power Measurement2/2 -> Q/1
  PS-Simulink Converter3/1 -> RMS Measurement3/1, Display4/1, Scope8/1
  Power Measurement2/1 -> Q1/1, Display5/1, Scope10/1
  RMS Measurement2/1 -> Scope7/1, Display3/1, Power Measurement2/1
  PS-Simulink Converter2/1 -> RMS Measurement2/1, Scope6/1
  RMS Measurement3/1 -> Power Measurement2/2, Scope9/1
  connections:
  PS-Simulink Converter3/LConn1 -- input1/RConn1
  PS-Simulink Converter2/LConn1 -- input/RConn1

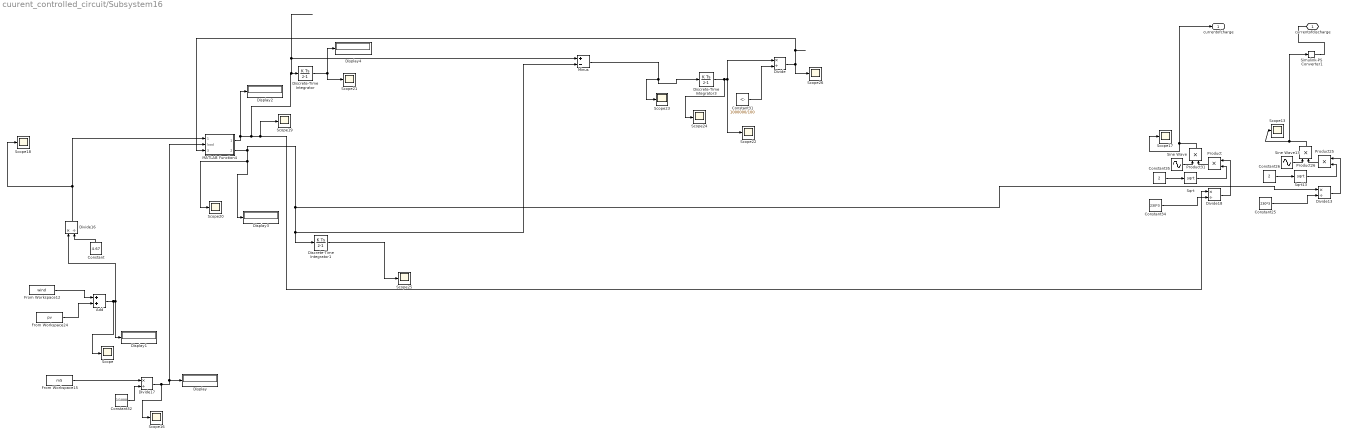
== system cuurent_controlled_circuit/Subsystem16 ==
  Add : Sum
  Constant : Constant  Value=4.67
  Constant25 : Constant  Value=230*3
  Constant26 : Constant  Value=2
  Constant31 : Constant  Value=1000000/100
  Constant32 : Constant  Value=1/1000
  Constant34 : Constant  Value=230*3
  Constant35 : Constant  Value=2
  Discrete-Time Integrator : DiscreteIntegrator  ICPrevOutput=DiscIntNeverNeededParam  ICPrevScaledInput=DiscIntNeverNeededParam
  Discrete-Time Integrator1 : DiscreteIntegrator  ICPrevOutput=DiscIntNeverNeededParam  ICPrevScaledInput=DiscIntNeverNeededParam
  Discrete-Time Integrator3 : DiscreteIntegrator  InitialCondition=500000  ICPrevOutput=DiscIntNeverNeededParam  ICPrevScaledInput=DiscIntNeverNeededParam
  Display{,1..4} (5 alike) : Display
  Divide{,13,16..18} (5 alike) : Product  Inputs=*/
  From Workspace12 : FromWorkspace  VariableName=wind  SampleTime=1  Interpolate=off  OutputAfterFinalValue=Holding final value
  From Workspace15 : FromWorkspace  VariableName=m5  SampleTime=1  Interpolate=off  OutputAfterFinalValue=Holding final value
  From Workspace24 : FromWorkspace  VariableName=pv  SampleTime=1  Interpolate=off  OutputAfterFinalValue=Holding final value
  MATLAB Function4 : MATLAB Function  TreatAsAtomicUnit=on
  Minus : Sum  Inputs=+-
  Product{,25..26,31} (4 alike) : Product
  Scope{,13,16..26} (13 alike) : Scope
  Simulink-PS Converter1 : nesl_utility/Simulink-PS Converter  PhysicalDomain=network_engine_domain  SubClassName=ps_input  LeftPortType=input  RightPortType=output  PseudoPeriodic=off  Frequencies=[]  NoiseDistribution=none  NoiseParameters=[]  Unit=1  AffineConversion=off  FilteringAndDerivatives=provide  SimscapeFilterOrder=1  InputFilterTimeConstant=0.001  UdotUserProvided=0
      settings: SourceProductBaseCode=SS,PW,VE
  Sine Wave : Sin  Frequency=314.6  Phase=120  SampleTime=0
  Sine Wave13 : Sin  Frequency=314.6  Phase=120  SampleTime=0
  Sqrt : Sqrt
  Sqrt13 : Sqrt
  currentofdischarge : PMIOPort  Side=Right
  currentofcharge : Outport
  wires:
  MATLAB Function4/1(charge) -> Minus/1, Discrete-Time Integrator/1, Divide18/1, Scope19/1, Display2/1
  MATLAB Function4/2(discharge) -> Divide13/1, Minus/2, Discrete-Time Integrator1/1, Scope20/1, Display3/1
  Divide/1 -> MATLAB Function4/3(batterycharge), Scope26/1
  Sine Wave13/1 -> Product26/1
  Product26/1 -> Simulink-PS Converter1/1, Scope13/1
  Discrete-Time Integrator/1 -> Display4/1, Scope21/1
  From Workspace24/1 -> Add/2
  Constant35/1 -> Sqrt/1
  Constant26/1 -> Sqrt13/1
  Product31/1 -> currentofcharge/1, Scope17/1
  Divide17/1 -> Scope16/1, MATLAB Function4/2(load), Display/1
  Divide13/1 -> Product25/1
  Add/1 -> Scope/1, Divide16/1, Display1/1
  Constant31/1 -> Divide/2
  Discrete-Time Integrator1/1 -> Scope25/1
  From Workspace15/1 -> Divide17/1
  Constant32/1 -> Divide17/2
  Minus/1 -> Discrete-Time Integrator3/1, Scope23/1
  Divide18/1 -> Product/1
  Discrete-Time Integrator3/1 -> Scope24/1, Divide/1, Scope22/1
  Product/1 -> Product31/2
  Product25/1 -> Product26/2
  Constant25/1 -> Divide13/2
  Constant/1 -> Divide16/2
  Divide16/1 -> Scope18/1, MATLAB Function4/1(pvandwind)
  Sine Wave/1 -> Product31/1
  Constant34/1 -> Divide18/2
  Sqrt/1 -> Product/2
  Sqrt13/1 -> Product25/2
  From Workspace12/1 -> Add/1
  connections:
  Simulink-PS Converter1/RConn1 -- currentofdischarge/RConn1

== system cuurent_controlled_circuit/Subsystem17 ==
  Display3 : Display
  Display4 : Display
  Display5 : Display
  PS-Simulink Converter2 : nesl_utility/PS-Simulink Converter  PhysicalDomain=network_engine_domain  SubClassName=ps_output  LeftPortType=input  RightPortType=output  PseudoPeriodic=off  Frequencies=[]  VectorFormat=inherit  Unit=inherit  AffineConversion=off
      settings: SourceProductBaseCode=SS,PW,VE
  PS-Simulink Converter3 : nesl_utility/PS-Simulink Converter  PhysicalDomain=network_engine_domain  SubClassName=ps_output  LeftPortType=input  RightPortType=output  PseudoPeriodic=off  Frequencies=[]  VectorFormat=inherit  Unit=inherit  AffineConversion=off
      settings: SourceProductBaseCode=SS,PW,VE
  Power Measurement2 : eePowerMeasurement/Power Measurement  LabelModeActiveChoice=Continuous  F=50  K=[0 1 2 3]  Ts=0
      settings: SourceProductBaseCode=PS
  RMS Measurement2 : eeRmsMeasurement/RMS Measurement  LabelModeActiveChoice=Total  F=50  SpecifyHarmonics=off  K=[0 1 2]  Ts=0
      settings: SourceProductBaseCode=PS
  RMS Measurement3 : eeRmsMeasurement/RMS Measurement  LabelModeActiveChoice=Total  F=50  SpecifyHarmonics=off  K=[0 1 2]  Ts=0
      settings: SourceProductBaseCode=PS
  Scope{6..10} (5 alike) : Scope
  input : PMIOPort  Side=Left
  input1 : PMIOPort  Port=2  Side=Left
  Q : Outport
  Q1 : Outport  Port=2
  wires:
  Power Measurement2/2 -> Q/1
  PS-Simulink Converter3/1 -> RMS Measurement3/1, Display4/1, Scope8/1
  Power Measurement2/1 -> Q1/1, Display5/1, Scope10/1
  RMS Measurement2/1 -> Scope7/1, Display3/1, Power Measurement2/1
  PS-Simulink Converter2/1 -> RMS Measurement2/1, Scope6/1
  RMS Measurement3/1 -> Power Measurement2/2, Scope9/1
  connections:
  PS-Simulink Converter3/LConn1 -- input1/RConn1
  PS-Simulink Converter2/LConn1 -- input/RConn1

== system cuurent_controlled_circuit/Subsystem18 ==
  Display3 : Display
  Display4 : Display
  Display5 : Display
  PS-Simulink Converter2 : nesl_utility/PS-Simulink Converter  PhysicalDomain=network_engine_domain  SubClassName=ps_output  LeftPortType=input  RightPortType=output  PseudoPeriodic=off  Frequencies=[]  VectorFormat=inherit  Unit=inherit  AffineConversion=off
      settings: SourceProductBaseCode=SS,PW,VE
  PS-Simulink Converter3 : nesl_utility/PS-Simulink Converter  PhysicalDomain=network_engine_domain  SubClassName=ps_output  LeftPortType=input  RightPortType=output  PseudoPeriodic=off  Frequencies=[]  VectorFormat=inherit  Unit=inherit  AffineConversion=off
      settings: SourceProductBaseCode=SS,PW,VE
  Power Measurement2 : eePowerMeasurement/Power Measurement  LabelModeActiveChoice=Continuous  F=50  K=[0 1 2 3]  Ts=0
      settings: SourceProductBaseCode=PS
  RMS Measurement2 : eeRmsMeasurement/RMS Measurement  LabelModeActiveChoice=Total  F=50  SpecifyHarmonics=off  K=[0 1 2]  Ts=0
      settings: SourceProductBaseCode=PS
  RMS Measurement3 : eeRmsMeasurement/RMS Measurement  LabelModeActiveChoice=Total  F=50  SpecifyHarmonics=off  K=[0 1 2]  Ts=0
      settings: SourceProductBaseCode=PS
  Scope{6..10} (5 alike) : Scope
  input : PMIOPort  Side=Left
  input1 : PMIOPort  Port=2  Side=Left
  Q : Outport
  Q1 : Outport  Port=2
  wires:
  Power Measurement2/2 -> Q/1
  PS-Simulink Converter3/1 -> RMS Measurement3/1, Display4/1, Scope8/1
  Power Measurement2/1 -> Q1/1, Display5/1, Scope10/1
  RMS Measurement2/1 -> Scope7/1, Display3/1, Power Measurement2/1
  PS-Simulink Converter2/1 -> RMS Measurement2/1, Scope6/1
  RMS Measurement3/1 -> Power Measurement2/2, Scope9/1
  connections:
  PS-Simulink Converter3/LConn1 -- input1/RConn1
  PS-Simulink Converter2/LConn1 -- input/RConn1

== system cuurent_controlled_circuit/Subsystem19 ==
  Add : Sum
  Battery Management System : MATLAB Function  TreatAsAtomicUnit=on
  Constant : Constant  Value=4.67
  Constant25 : Constant  Value=230*3
  Constant26 : Constant  Value=2
  Constant31 : Constant  Value=1000000/100
  Constant32 : Constant  Value=1/1000
  Constant34 : Constant  Value=230*3
  Constant35 : Constant  Value=2
  Discrete-Time Integrator3 : DiscreteIntegrator  InitialCondition=500000  ICPrevOutput=DiscIntNeverNeededParam  ICPrevScaledInput=DiscIntNeverNeededParam
  Divide{,13,16..18} (5 alike) : Product  Inputs=*/
  From Workspace12 : FromWorkspace  VariableName=wind  SampleTime=1  Interpolate=off  OutputAfterFinalValue=Holding final value
  From Workspace15 : FromWorkspace  VariableName=m5  SampleTime=1  Interpolate=off  OutputAfterFinalValue=Holding final value
  From Workspace24 : FromWorkspace  VariableName=pv  SampleTime=1  Interpolate=off  OutputAfterFinalValue=Holding final value
  Minus : Sum  Inputs=+-
  Product{,25..26,31} (4 alike) : Product
  Simulink-PS Converter1 : nesl_utility/Simulink-PS Converter  PhysicalDomain=network_engine_domain  SubClassName=ps_input  LeftPortType=input  RightPortType=output  PseudoPeriodic=off  Frequencies=[]  NoiseDistribution=none  NoiseParameters=[]  Unit=1  AffineConversion=off  FilteringAndDerivatives=provide  SimscapeFilterOrder=1  InputFilterTimeConstant=0.001  UdotUserProvided=0
      settings: SourceProductBaseCode=SS,PW,VE
  Sine Wave : Sin  Frequency=314.6  SampleTime=0
  Sine Wave13 : Sin  Frequency=314.6  SampleTime=0
  Sqrt : Sqrt
  Sqrt13 : Sqrt
  currentofdischarge : PMIOPort  Side=Right
  currentofcharge : Outport
  Input : Outport  Port=2
  wires:
  Battery Management System/1(charge) -> Divide18/1, Minus/1
  Battery Management System/2(discharge) -> Divide13/1, Minus/2
  Sine Wave13/1 -> Product26/1
  Product26/1 -> Simulink-PS Converter1/1
  From Workspace24/1 -> Add/2
  Constant35/1 -> Sqrt/1
  Constant26/1 -> Sqrt13/1
  Product31/1 -> currentofcharge/1
  Divide17/1 -> Battery Management System/2(load)
  Divide13/1 -> Product25/1
  Add/1 -> Divide16/1
  Constant31/1 -> Divide/2
  From Workspace15/1 -> Divide17/1
  Constant32/1 -> Divide17/2
  Minus/1 -> Discrete-Time Integrator3/1
  Divide18/1 -> Product/1
  Discrete-Time Integrator3/1 -> Divide/1
  Product/1 -> Product31/2
  Product25/1 -> Product26/2
  Constant25/1 -> Divide13/2
  Constant/1 -> Divide16/2
  Divide16/1 -> Battery Management System/1(pvandwind)
  Sine Wave/1 -> Product31/1
  Constant34/1 -> Divide18/2
  Sqrt/1 -> Product/2
  Sqrt13/1 -> Product25/2
  From Workspace12/1 -> Add/1
  Divide/1 -> Battery Management System/3(batterycharge), Input/1
  connections:
  Simulink-PS Converter1/RConn1 -- currentofdischarge/RConn1
